simulink model "A3VSM390_2023b"  (R2023b)
settings: Solver=ode14x  StartTime=0  StopTime=Sim.tend  FixedStep=0.000125  RelTol=4e-4
values from neighbouring files (symbols this model uses):
  center_line_status = parameterset.center_line_status    [sim3run_390.m]
  ControlSampleTime = 1/8000    (= 0.000125)    [sim3run_390.m]
  k_ring1 = 1    [sim3run_390.m]
  k_ring2 = 1    [sim3run_390.m]
  load_start_factor = 1    [prm3var_390.m]    (also in simu3_826.m = 0.9; simu3_827.m = 0.9)
  lower_line_status = parameterset.lower_line_status    [sim3run_390.m]
  mZC = 3    [sim3run_390.m]
undefined symbols (not defined in the file or in its folder): Event, General, InfBus, Li, parameterset, prm_vsm, pu_vsm, TrG, VSM
libraries: fl_lib x92, nesl_utility x69, ee_lib x36, spsPower3phInstantaneousLib x5, simulink x2, eeTransforms x1
(part 2 of 3)

== system A3VSM390_2023b/Inverter AverageMdl LC SimScape0/Modul F30 fixed DC voltage Average SimScape ==
  ctrl : Inport
  Phase Splitter : ee_lib/Connectors & References/Phase Splitter
  Rate Transition : RateTransition  Integrity=off  InitialCondition=-1  OutPortSampleTime=ControlSampleTime
  ctrlSelect3 : Subsystem
  measMerge3 : Subsystem
  simscape_bridgefilter_aca : Subsystem  mask{L1=L1, R_L1=R_L1, C1=C1, R_C1=R_C1}
      mask prompts: L1 "Inductance L1 [H]"; R_L1 "Resistance of L1 [Ohm]"; C1 "Capacitance C1 [F]"; R_C1 "Parallel resistance of C1 [Ohm]"
      mask DialogControl LC Prompt: LC(L)(C)
      mask DialogControl GrpLC Prompt: LC(L)(C)-Filter
  simscape_bridgefilter_aca1 : Subsystem  mask{L1=L1, R_L1=R_L1, C1=C1, R_C1=R_C1}
      mask prompts: L1 "Inductance L1 [H]"; R_L1 "Resistance of L1 [Ohm]"; C1 "Capacitance C1 [F]"; R_C1 "Parallel resistance of C1 [Ohm]"
      mask DialogControl LC Prompt: LC(L)(C)
      mask DialogControl GrpLC Prompt: LC(L)(C)-Filter
  simscape_bridgefilter_aca2 : Subsystem  mask{L1=L1, R_L1=R_L1, C1=C1, R_C1=R_C1}
      mask prompts: L1 "Inductance L1 [H]"; R_L1 "Resistance of L1 [Ohm]"; C1 "Capacitance C1 [F]"; R_C1 "Parallel resistance of C1 [Ohm]"
      mask DialogControl LC Prompt: LC(L)(C)
      mask DialogControl GrpLC Prompt: LC(L)(C)-Filter
  N : PMIOPort  Side=Left
  ABC : PMIOPort  Port=2  Side=Right
  meas : Outport  VectorParamsAs1DForOutWhenUnconnected=off
  wires:
  measMerge3/1(meas) -> Rate Transition/1
  ctrlSelect3/1(ctrl1) -> simscape_bridgefilter_aca/1(ctrl)
  [ctrl3] -> simscape_bridgefilter_aca2/1(ctrl)
  [ctrl2] -> simscape_bridgefilter_aca1/1(ctrl)
  ctrlSelect3/2(ctrl2) -> [ctrl2]
  ctrlSelect3/3(ctrl3) -> [ctrl3]
  ctrl/1 -> ctrlSelect3/1(ctrl)
  [meas2] -> measMerge3/2(meas2)
  simscape_bridgefilter_aca2/1(meas) -> [meas3]
  simscape_bridgefilter_aca1/1(meas) -> [meas2]
  [meas3] -> measMerge3/3(meas3)
  simscape_bridgefilter_aca/1(meas) -> measMerge3/1(meas1)
  Rate Transition/1 -> meas/1
  connections:
  simscape_bridgefilter_aca/LConn2 -- simscape_bridgefilter_aca1/LConn2 -- simscape_bridgefilter_aca2/LConn2 -- N/RConn1
  simscape_bridgefilter_aca/RConn1 -- simscape_bridgefilter_aca2/RConn1 -- simscape_bridgefilter_aca1/RConn1
  simscape_bridgefilter_aca2/LConn1 -- Phase Splitter/RConn3
  ABC/RConn1 -- Phase Splitter/LConn1
  Phase Splitter/RConn1 -- simscape_bridgefilter_aca/LConn1
  simscape_bridgefilter_aca1/LConn1 -- Phase Splitter/RConn2

== system A3VSM390_2023b/Inverter AverageMdl LC SimScape1/Modul F30 fixed DC voltage Average SimScape ==
  ctrl : Inport
  Phase Splitter : ee_lib/Connectors & References/Phase Splitter
  Rate Transition : RateTransition  Integrity=off  InitialCondition=-1  OutPortSampleTime=ControlSampleTime
  ctrlSelect3 : Subsystem
  measMerge3 : Subsystem
  simscape_bridgefilter_aca : Subsystem  mask{L1=L1, R_L1=R_L1, C1=C1, R_C1=R_C1}
      mask prompts: L1 "Inductance L1 [H]"; R_L1 "Resistance of L1 [Ohm]"; C1 "Capacitance C1 [F]"; R_C1 "Parallel resistance of C1 [Ohm]"
      mask DialogControl LC Prompt: LC(L)(C)
      mask DialogControl GrpLC Prompt: LC(L)(C)-Filter
  simscape_bridgefilter_aca1 : Subsystem  mask{L1=L1, R_L1=R_L1, C1=C1, R_C1=R_C1}
      mask prompts: L1 "Inductance L1 [H]"; R_L1 "Resistance of L1 [Ohm]"; C1 "Capacitance C1 [F]"; R_C1 "Parallel resistance of C1 [Ohm]"
      mask DialogControl LC Prompt: LC(L)(C)
      mask DialogControl GrpLC Prompt: LC(L)(C)-Filter
  simscape_bridgefilter_aca2 : Subsystem  mask{L1=L1, R_L1=R_L1, C1=C1, R_C1=R_C1}
      mask prompts: L1 "Inductance L1 [H]"; R_L1 "Resistance of L1 [Ohm]"; C1 "Capacitance C1 [F]"; R_C1 "Parallel resistance of C1 [Ohm]"
      mask DialogControl LC Prompt: LC(L)(C)
      mask DialogControl GrpLC Prompt: LC(L)(C)-Filter
  N : PMIOPort  Side=Left
  ABC : PMIOPort  Port=2  Side=Right
  meas : Outport  VectorParamsAs1DForOutWhenUnconnected=off
  wires:
  measMerge3/1(meas) -> Rate Transition/1
  ctrlSelect3/1(ctrl1) -> simscape_bridgefilter_aca/1(ctrl)
  [ctrl3] -> simscape_bridgefilter_aca2/1(ctrl)
  [ctrl2] -> simscape_bridgefilter_aca1/1(ctrl)
  ctrlSelect3/2(ctrl2) -> [ctrl2]
  ctrlSelect3/3(ctrl3) -> [ctrl3]
  ctrl/1 -> ctrlSelect3/1(ctrl)
  [meas2] -> measMerge3/2(meas2)
  simscape_bridgefilter_aca2/1(meas) -> [meas3]
  simscape_bridgefilter_aca1/1(meas) -> [meas2]
  [meas3] -> measMerge3/3(meas3)
  simscape_bridgefilter_aca/1(meas) -> measMerge3/1(meas1)
  Rate Transition/1 -> meas/1
  connections:
  simscape_bridgefilter_aca/LConn2 -- simscape_bridgefilter_aca1/LConn2 -- simscape_bridgefilter_aca2/LConn2 -- N/RConn1
  simscape_bridgefilter_aca/RConn1 -- simscape_bridgefilter_aca2/RConn1 -- simscape_bridgefilter_aca1/RConn1
  simscape_bridgefilter_aca2/LConn1 -- Phase Splitter/RConn3
  ABC/RConn1 -- Phase Splitter/LConn1
  Phase Splitter/RConn1 -- simscape_bridgefilter_aca/LConn1
  simscape_bridgefilter_aca1/LConn1 -- Phase Splitter/RConn2

== system A3VSM390_2023b/Inverter AverageMdl LC SimScape2/Modul F30 fixed DC voltage Average SimScape ==
  ctrl : Inport
  Phase Splitter : ee_lib/Connectors & References/Phase Splitter
  Rate Transition : RateTransition  Integrity=off  InitialCondition=-1  OutPortSampleTime=ControlSampleTime
  ctrlSelect3 : Subsystem
  measMerge3 : Subsystem
  simscape_bridgefilter_aca : Subsystem  mask{L1=L1, R_L1=R_L1, C1=C1, R_C1=R_C1}
      mask prompts: L1 "Inductance L1 [H]"; R_L1 "Resistance of L1 [Ohm]"; C1 "Capacitance C1 [F]"; R_C1 "Parallel resistance of C1 [Ohm]"
      mask DialogControl LC Prompt: LC(L)(C)
      mask DialogControl GrpLC Prompt: LC(L)(C)-Filter
  simscape_bridgefilter_aca1 : Subsystem  mask{L1=L1, R_L1=R_L1, C1=C1, R_C1=R_C1}
      mask prompts: L1 "Inductance L1 [H]"; R_L1 "Resistance of L1 [Ohm]"; C1 "Capacitance C1 [F]"; R_C1 "Parallel resistance of C1 [Ohm]"
      mask DialogControl LC Prompt: LC(L)(C)
      mask DialogControl GrpLC Prompt: LC(L)(C)-Filter
  simscape_bridgefilter_aca2 : Subsystem  mask{L1=L1, R_L1=R_L1, C1=C1, R_C1=R_C1}
      mask prompts: L1 "Inductance L1 [H]"; R_L1 "Resistance of L1 [Ohm]"; C1 "Capacitance C1 [F]"; R_C1 "Parallel resistance of C1 [Ohm]"
      mask DialogControl LC Prompt: LC(L)(C)
      mask DialogControl GrpLC Prompt: LC(L)(C)-Filter
  N : PMIOPort  Side=Left
  ABC : PMIOPort  Port=2  Side=Right
  meas : Outport  VectorParamsAs1DForOutWhenUnconnected=off
  wires:
  measMerge3/1(meas) -> Rate Transition/1
  ctrlSelect3/1(ctrl1) -> simscape_bridgefilter_aca/1(ctrl)
  [ctrl3] -> simscape_bridgefilter_aca2/1(ctrl)
  [ctrl2] -> simscape_bridgefilter_aca1/1(ctrl)
  ctrlSelect3/2(ctrl2) -> [ctrl2]
  ctrlSelect3/3(ctrl3) -> [ctrl3]
  ctrl/1 -> ctrlSelect3/1(ctrl)
  [meas2] -> measMerge3/2(meas2)
  simscape_bridgefilter_aca2/1(meas) -> [meas3]
  simscape_bridgefilter_aca1/1(meas) -> [meas2]
  [meas3] -> measMerge3/3(meas3)
  simscape_bridgefilter_aca/1(meas) -> measMerge3/1(meas1)
  Rate Transition/1 -> meas/1
  connections:
  simscape_bridgefilter_aca/LConn2 -- simscape_bridgefilter_aca1/LConn2 -- simscape_bridgefilter_aca2/LConn2 -- N/RConn1
  simscape_bridgefilter_aca/RConn1 -- simscape_bridgefilter_aca2/RConn1 -- simscape_bridgefilter_aca1/RConn1
  simscape_bridgefilter_aca2/LConn1 -- Phase Splitter/RConn3
  ABC/RConn1 -- Phase Splitter/LConn1
  Phase Splitter/RConn1 -- simscape_bridgefilter_aca/LConn1
  simscape_bridgefilter_aca1/LConn1 -- Phase Splitter/RConn2

== system A3VSM390_2023b/Subsystem2/I_PhN1 ==
  In1 : Inport
  Abs : Abs  SaturateOnIntegerOverflow=off
  Demux : Demux  Outputs=2
  PhN->ab0 : Subsystem
      mask Display:
      | plot([0 1], [0,1])
      | plot([0.1 0.25 0.4 0.25 0.25], [0.5 0.6 0.5 0.6 0.8]) % Stern
      | text(0.05,1,'PhN','VerticalAlignment','Top')
      | text(0.55, 0.3,'\alpha\beta0','texmode','on')
  Real-Imag to Complex : RealImagToComplex
  Selector4 : Selector  InputPortWidth=3  IndexOptions=Index vector (dialog)  Indices=[1 2]  OutputSizes=1
  Out1 : Outport  VectorParamsAs1DForOutWhenUnconnected=off
  wires:
  Demux/1 -> Real-Imag to Complex/1
  PhN->ab0/1(ab0) -> Selector4/1
  Selector4/1 -> Demux/1
  Real-Imag to Complex/1 -> Abs/1
  Demux/2 -> Real-Imag to Complex/2
  Abs/1 -> Out1/1
  In1/1 -> PhN->ab0/1(PhN)

== system A3VSM390_2023b/Subsystem2/I_PhN2 ==
  In1 : Inport
  Abs : Abs  SaturateOnIntegerOverflow=off
  Demux : Demux  Outputs=2
  PhN->ab0 : Subsystem
      mask Display:
      | plot([0 1], [0,1])
      | plot([0.1 0.25 0.4 0.25 0.25], [0.5 0.6 0.5 0.6 0.8]) % Stern
      | text(0.05,1,'PhN','VerticalAlignment','Top')
      | text(0.55, 0.3,'\alpha\beta0','texmode','on')
  Real-Imag to Complex : RealImagToComplex
  Selector4 : Selector  InputPortWidth=3  IndexOptions=Index vector (dialog)  Indices=[1 2]  OutputSizes=1
  Out1 : Outport  VectorParamsAs1DForOutWhenUnconnected=off
  wires:
  Demux/1 -> Real-Imag to Complex/1
  PhN->ab0/1(ab0) -> Selector4/1
  Selector4/1 -> Demux/1
  Real-Imag to Complex/1 -> Abs/1
  Demux/2 -> Real-Imag to Complex/2
  Abs/1 -> Out1/1
  In1/1 -> PhN->ab0/1(PhN)

== system A3VSM390_2023b/Subsystem2/I_PhN3 ==
  In1 : Inport
  Abs : Abs  SaturateOnIntegerOverflow=off
  Demux : Demux  Outputs=2
  PhN->ab0 : Subsystem
      mask Display:
      | plot([0 1], [0,1])
      | plot([0.1 0.25 0.4 0.25 0.25], [0.5 0.6 0.5 0.6 0.8]) % Stern
      | text(0.05,1,'PhN','VerticalAlignment','Top')
      | text(0.55, 0.3,'\alpha\beta0','texmode','on')
  Real-Imag to Complex : RealImagToComplex
  Selector4 : Selector  InputPortWidth=3  IndexOptions=Index vector (dialog)  Indices=[1 2]  OutputSizes=1
  Out1 : Outport  VectorParamsAs1DForOutWhenUnconnected=off
  wires:
  Demux/1 -> Real-Imag to Complex/1
  PhN->ab0/1(ab0) -> Selector4/1
  Selector4/1 -> Demux/1
  Real-Imag to Complex/1 -> Abs/1
  Demux/2 -> Real-Imag to Complex/2
  Abs/1 -> Out1/1
  In1/1 -> PhN->ab0/1(PhN)

== system A3VSM390_2023b/Subsystem2/I_PhN4 ==
  In1 : Inport
  Abs : Abs  SaturateOnIntegerOverflow=off
  Demux : Demux  Outputs=2
  PhN->ab0 : Subsystem
      mask Display:
      | plot([0 1], [0,1])
      | plot([0.1 0.25 0.4 0.25 0.25], [0.5 0.6 0.5 0.6 0.8]) % Stern
      | text(0.05,1,'PhN','VerticalAlignment','Top')
      | text(0.55, 0.3,'\alpha\beta0','texmode','on')
  Real-Imag to Complex : RealImagToComplex
  Selector4 : Selector  InputPortWidth=3  IndexOptions=Index vector (dialog)  Indices=[1 2]  OutputSizes=1
  Out1 : Outport  VectorParamsAs1DForOutWhenUnconnected=off
  wires:
  In1/1 -> PhN->ab0/1(PhN)
  Abs/1 -> Out1/1
  Demux/2 -> Real-Imag to Complex/2
  Real-Imag to Complex/1 -> Abs/1
  Selector4/1 -> Demux/1
  PhN->ab0/1(ab0) -> Selector4/1
  Demux/1 -> Real-Imag to Complex/1

== system A3VSM390_2023b/Subsystem2/I_PhN5 ==
  In1 : Inport
  Abs : Abs  SaturateOnIntegerOverflow=off
  Demux : Demux  Outputs=2
  PhN->ab0 : Subsystem
      mask Display:
      | plot([0 1], [0,1])
      | plot([0.1 0.25 0.4 0.25 0.25], [0.5 0.6 0.5 0.6 0.8]) % Stern
      | text(0.05,1,'PhN','VerticalAlignment','Top')
      | text(0.55, 0.3,'\alpha\beta0','texmode','on')
  Real-Imag to Complex : RealImagToComplex
  Selector4 : Selector  InputPortWidth=3  IndexOptions=Index vector (dialog)  Indices=[1 2]  OutputSizes=1
  Out1 : Outport  VectorParamsAs1DForOutWhenUnconnected=off
  wires:
  Demux/1 -> Real-Imag to Complex/1
  PhN->ab0/1(ab0) -> Selector4/1
  Selector4/1 -> Demux/1
  Real-Imag to Complex/1 -> Abs/1
  Demux/2 -> Real-Imag to Complex/2
  Abs/1 -> Out1/1
  In1/1 -> PhN->ab0/1(PhN)

== system A3VSM390_2023b/Subsystem2/V_PhN ==
  In1 : Inport
  Abs : Abs  SaturateOnIntegerOverflow=off
  Demux : Demux  Outputs=2
  PhN->ab0 : Subsystem
      mask Display:
      | plot([0 1], [0,1])
      | plot([0.1 0.25 0.4 0.25 0.25], [0.5 0.6 0.5 0.6 0.8]) % Stern
      | text(0.05,1,'PhN','VerticalAlignment','Top')
      | text(0.55, 0.3,'\alpha\beta0','texmode','on')
  Real-Imag to Complex : RealImagToComplex
  Selector4 : Selector  InputPortWidth=3  IndexOptions=Index vector (dialog)  Indices=[1 2]  OutputSizes=1
  Out1 : Outport  VectorParamsAs1DForOutWhenUnconnected=off
  wires:
  In1/1 -> PhN->ab0/1(PhN)
  Abs/1 -> Out1/1
  Demux/2 -> Real-Imag to Complex/2
  Real-Imag to Complex/1 -> Abs/1
  Selector4/1 -> Demux/1
  PhN->ab0/1(ab0) -> Selector4/1
  Demux/1 -> Real-Imag to Complex/1

== system A3VSM390_2023b/Subsystem2/V_PhN1 ==
  In1 : Inport
  Abs : Abs  SaturateOnIntegerOverflow=off
  Demux : Demux  Outputs=2
  PhN->ab0 : Subsystem
      mask Display:
      | plot([0 1], [0,1])
      | plot([0.1 0.25 0.4 0.25 0.25], [0.5 0.6 0.5 0.6 0.8]) % Stern
      | text(0.05,1,'PhN','VerticalAlignment','Top')
      | text(0.55, 0.3,'\alpha\beta0','texmode','on')
  Real-Imag to Complex : RealImagToComplex
  Selector4 : Selector  InputPortWidth=3  IndexOptions=Index vector (dialog)  Indices=[1 2]  OutputSizes=1
  Out1 : Outport  VectorParamsAs1DForOutWhenUnconnected=off
  wires:
  Demux/1 -> Real-Imag to Complex/1
  PhN->ab0/1(ab0) -> Selector4/1
  Selector4/1 -> Demux/1
  Real-Imag to Complex/1 -> Abs/1
  Demux/2 -> Real-Imag to Complex/2
  Abs/1 -> Out1/1
  In1/1 -> PhN->ab0/1(PhN)

== system A3VSM390_2023b/Subsystem2/V_PhN2 ==
  In1 : Inport
  Abs : Abs  SaturateOnIntegerOverflow=off
  Demux : Demux  Outputs=2
  PhN->ab0 : Subsystem
      mask Display:
      | plot([0 1], [0,1])
      | plot([0.1 0.25 0.4 0.25 0.25], [0.5 0.6 0.5 0.6 0.8]) % Stern
      | text(0.05,1,'PhN','VerticalAlignment','Top')
      | text(0.55, 0.3,'\alpha\beta0','texmode','on')
  Real-Imag to Complex : RealImagToComplex
  Selector4 : Selector  InputPortWidth=3  IndexOptions=Index vector (dialog)  Indices=[1 2]  OutputSizes=1
  Out1 : Outport  VectorParamsAs1DForOutWhenUnconnected=off
  wires:
  Demux/1 -> Real-Imag to Complex/1
  PhN->ab0/1(ab0) -> Selector4/1
  Selector4/1 -> Demux/1
  Real-Imag to Complex/1 -> Abs/1
  Demux/2 -> Real-Imag to Complex/2
  Abs/1 -> Out1/1
  In1/1 -> PhN->ab0/1(PhN)

== system A3VSM390_2023b/Subsystem2/V_PhN3 ==
  In1 : Inport
  Abs : Abs  SaturateOnIntegerOverflow=off
  Demux : Demux  Outputs=2
  PhN->ab0 : Subsystem
      mask Display:
      | plot([0 1], [0,1])
      | plot([0.1 0.25 0.4 0.25 0.25], [0.5 0.6 0.5 0.6 0.8]) % Stern
      | text(0.05,1,'PhN','VerticalAlignment','Top')
      | text(0.55, 0.3,'\alpha\beta0','texmode','on')
  Real-Imag to Complex : RealImagToComplex
  Selector4 : Selector  InputPortWidth=3  IndexOptions=Index vector (dialog)  Indices=[1 2]  OutputSizes=1
  Out1 : Outport  VectorParamsAs1DForOutWhenUnconnected=off
  wires:
  Demux/1 -> Real-Imag to Complex/1
  PhN->ab0/1(ab0) -> Selector4/1
  Selector4/1 -> Demux/1
  Real-Imag to Complex/1 -> Abs/1
  Demux/2 -> Real-Imag to Complex/2
  Abs/1 -> Out1/1
  In1/1 -> PhN->ab0/1(PhN)

== system A3VSM390_2023b/Subsystem2/V_PhN4 ==
  In1 : Inport
  Abs : Abs  SaturateOnIntegerOverflow=off
  Demux : Demux  Outputs=2
  PhN->ab0 : Subsystem
      mask Display:
      | plot([0 1], [0,1])
      | plot([0.1 0.25 0.4 0.25 0.25], [0.5 0.6 0.5 0.6 0.8]) % Stern
      | text(0.05,1,'PhN','VerticalAlignment','Top')
      | text(0.55, 0.3,'\alpha\beta0','texmode','on')
  Real-Imag to Complex : RealImagToComplex
  Selector4 : Selector  InputPortWidth=3  IndexOptions=Index vector (dialog)  Indices=[1 2]  OutputSizes=1
  Out1 : Outport  VectorParamsAs1DForOutWhenUnconnected=off
  wires:
  Demux/1 -> Real-Imag to Complex/1
  PhN->ab0/1(ab0) -> Selector4/1
  Selector4/1 -> Demux/1
  Real-Imag to Complex/1 -> Abs/1
  Demux/2 -> Real-Imag to Complex/2
  Abs/1 -> Out1/1
  In1/1 -> PhN->ab0/1(PhN)

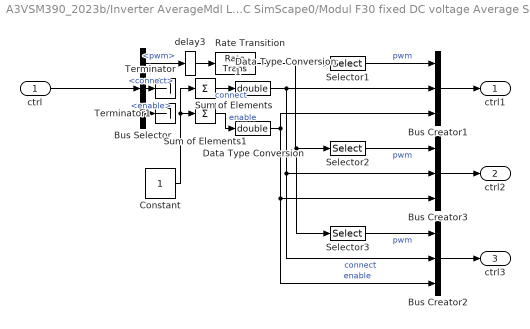
== system A3VSM390_2023b/Inverter AverageMdl LC SimScape0/Modul F30 fixed DC voltage Average SimScape/ctrlSelect3 ==
  ctrl : Inport
  Bus Creator1 : BusCreator  Inputs=3
  Bus Creator2 : BusCreator  Inputs=3
  Bus Creator3 : BusCreator  Inputs=3
  Bus Selector : BusSelector  OutputSignals=pwm,connect,enable
  Constant : Constant
  Data Type Conversion : DataTypeConversion  OutDataTypeStr=double  SaturateOnIntegerOverflow=off  RndMeth=Floor
  Data Type Conversion1 : DataTypeConversion  OutDataTypeStr=double  SaturateOnIntegerOverflow=off  RndMeth=Floor
  Rate Transition : RateTransition  Integrity=off  Deterministic=off  OutPortSampleTime=0
  Selector1 : Selector  InputPortWidth=3  IndexOptions=Index vector (dialog)  Indices=[1]  OutputSizes=1
  Selector2 : Selector  InputPortWidth=3  IndexOptions=Index vector (dialog)  Indices=2  OutputSizes=1
  Selector3 : Selector  InputPortWidth=3  IndexOptions=Index vector (dialog)  Indices=3  OutputSizes=1
  Sum of Elements : Sum  Inputs=+
  Sum of Elements1 : Sum  Inputs=+  SampleTime=ControlSampleTime
  Terminator : Terminator
  Terminator1 : Terminator
  delay3 : UnitDelay  SampleTime=-1  HasFrameUpgradeWarning=on
  ctrl1 : Outport  VectorParamsAs1DForOutWhenUnconnected=off
  ctrl2 : Outport  Port=2  VectorParamsAs1DForOutWhenUnconnected=off
  ctrl3 : Outport  Port=3  VectorParamsAs1DForOutWhenUnconnected=off
  wires:
  Rate Transition/1 -> Selector1/1, Selector3/1, Selector2/1
  Sum of Elements1/1 -> Data Type Conversion/1  "enable"
  Selector1/1 -> Bus Creator1/1  "pwm"
  Bus Creator3/1 -> ctrl2/1
  Selector2/1 -> Bus Creator3/1  "pwm"
  Sum of Elements/1 -> Data Type Conversion1/1  "connect"
  Bus Creator1/1 -> ctrl1/1
  ctrl/1 -> Bus Selector/1
  Bus Creator2/1 -> ctrl3/1
  Selector3/1 -> Bus Creator2/1  "pwm"
  Bus Selector/1 -> delay3/1  "<pwm>"
  Data Type Conversion/1 -> Bus Creator1/3, Bus Creator2/3, Bus Creator3/3  "enable"
  Data Type Conversion1/1 -> Bus Creator2/2, Bus Creator3/2, Bus Creator1/2  "connect"
  Constant/1 -> Sum of Elements1/1, Sum of Elements/1
  Bus Selector/2 -> Terminator/1  "<connect>"
  Bus Selector/3 -> Terminator1/1  "<enable>"
  delay3/1 -> Rate Transition/1

== system A3VSM390_2023b/Inverter AverageMdl LC SimScape0/Modul F30 fixed DC voltage Average SimScape/measMerge3 ==
  meas1 : Inport
  meas2 : Inport  Port=2
  meas3 : Inport  Port=3
  measMerge123 : Subsystem
  meas : Outport  VectorParamsAs1DForOutWhenUnconnected=off
  wires:
  meas3/1 -> measMerge123/3(meas3)
  meas2/1 -> measMerge123/2(meas2)
  measMerge123/1(meas) -> meas/1
  meas1/1 -> measMerge123/1(meas1)

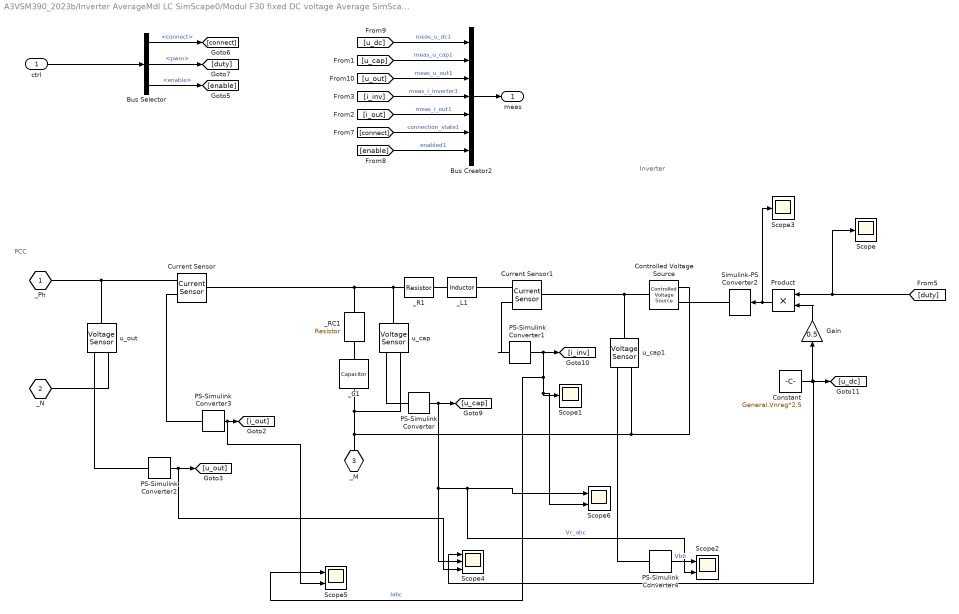
== system A3VSM390_2023b/Inverter AverageMdl LC SimScape0/Modul F30 fixed DC voltage Average SimScape/simscape_bridgefilter_aca ==
  note: Inverter
  note: PCC
  ctrl : Inport
  Bus Creator2 : BusCreator  Inputs=7
  Bus Selector : BusSelector  OutputSignals=connect,pwm,enable
  Constant : Constant  Value=General.Vnreg*2.5
  Controlled Voltage Source : fl_lib/Electrical/Electrical Sources/Controlled Voltage Source
  Current Sensor : fl_lib/Electrical/Electrical Sensors/Current Sensor
  Current Sensor1 : fl_lib/Electrical/Electrical Sensors/Current Sensor
  Gain : Gain  Gain=0.5
  PS-Simulink Converter{,1..4} (5 alike) : nesl_utility/PS-Simulink Converter  PhysicalDomain=network_engine_domain  SubClassName=ps_output  LeftPortType=input  RightPortType=output  PseudoPeriodic=off  Frequencies=[]  VectorFormat=1-D array  Unit=1  AffineConversion=off
  Product : Product
  Scope : Scope
  Scope1 : Scope
  Scope2 : Scope  NumInputPorts=2
  Scope3 : Scope
  Scope4 : Scope  NumInputPorts=3
  Scope5 : Scope  NumInputPorts=2
  Scope6 : Scope  NumInputPorts=2
  Simulink-PS Converter2 : nesl_utility/Simulink-PS Converter  PhysicalDomain=network_engine_domain  SubClassName=ps_input  LeftPortType=input  RightPortType=output  PseudoPeriodic=off  Frequencies=[]  NoiseDistribution=none  NoiseParameters=[]  Unit=1  AffineConversion=off  FilteringAndDerivatives=zero  SimscapeFilterOrder=1  InputFilterTimeConstant=0.001  UdotUserProvided=1
  _C1 : fl_lib/Electrical/Electrical Elements/Capacitor  c=C1 F  r=1e-6 Ohm  g=0 1/Ohm  i_specify=off  i_priority=None  i=0 A  i_nominal_specify=off  i_nominal_unit=A  i_nominal_value=1  v_specify=off  v_priority=None  v=0 V  v_nominal_specify=off  v_nominal_unit=V  v_nominal_value=1  vc_specify=off  vc_priority=None  vc=0 V  vc_nominal_specify=off  vc_nominal_unit=V  vc_nominal_value=1
  _L1 : fl_lib/Electrical/Electrical Elements/Inductor  l=L1 H  r=0 Ohm  g=1e-9 1/Ohm  i_specify=off  i_priority=None  i=0 A  i_nominal_specify=off  i_nominal_unit=A  i_nominal_value=1  v_specify=off  v_priority=None  v=0 V  v_nominal_specify=off  v_nominal_unit=V  v_nominal_value=1  i_L_specify=off  i_L_priority=None  i_L=0 A  i_L_nominal_specify=off  i_L_nominal_unit=A  i_L_nominal_value=1
  _R1 : fl_lib/Electrical/Electrical Elements/Resistor  R=R_L1 Ohm  i_specify=off  i_priority=None  i=0 A  i_nominal_specify=off  i_nominal_unit=A  i_nominal_value=1  v_specify=off  v_priority=None  v=0 V  v_nominal_specify=off  v_nominal_unit=V  v_nominal_value=1
  _RC1 : fl_lib/Electrical/Electrical Elements/Resistor  R=R_C1 Ohm  i_specify=off  i_priority=None  i=0 A  i_nominal_specify=off  i_nominal_unit=A  i_nominal_value=1  v_specify=off  v_priority=None  v=0 V  v_nominal_specify=off  v_nominal_unit=V  v_nominal_value=1
  u_cap : fl_lib/Electrical/Electrical Sensors/Voltage Sensor
  u_cap1 : fl_lib/Electrical/Electrical Sensors/Voltage Sensor
  u_out : fl_lib/Electrical/Electrical Sensors/Voltage Sensor
  _Ph : PMIOPort  Side=Left
  _N : PMIOPort  Port=2  Side=Left
  _M : PMIOPort  Port=3  Side=Right
  meas : Outport  VectorParamsAs1DForOutWhenUnconnected=off
  wires:
  Bus Selector/2 -> [duty]  "<pwm>"
  Bus Selector/1 -> [connect]  "<connect>"
  [connect] -> Bus Creator2/6  "connection_state1"
  ctrl/1 -> Bus Selector/1
  [i_out] -> Bus Creator2/5  "meas_i_out1"
  [i_inv] -> Bus Creator2/4  "meas_i_inverter1"
  [u_out] -> Bus Creator2/3  "meas_u_out1"
  [u_cap] -> Bus Creator2/2  "meas_u_cap1"
  Bus Selector/3 -> [enable]  "<enable>"
  [enable] -> Bus Creator2/7  "enabled1"
  Bus Creator2/1 -> meas/1
  [u_dc] -> Bus Creator2/1  "meas_u_dc1"
  PS-Simulink Converter/1 -> Scope2/2, Scope6/1, Scope4/2, [u_cap]  "Vc_abc"
  PS-Simulink Converter1/1 -> Scope5/1, Scope6/2, Scope1/1, [i_inv]  "Iabc"
  PS-Simulink Converter2/1 -> Scope4/3, [u_out]
  PS-Simulink Converter3/1 -> Scope5/2, [i_out]
  Product/1 -> Scope3/1, Simulink-PS Converter2/1
  Constant/1 -> Scope4/1, [u_dc], Gain/1
  [duty] -> Scope/1, Product/1
  Gain/1 -> Product/2
  PS-Simulink Converter4/1 -> Scope2/1  "Vb6"
  connections:
  _R1/RConn1 -- _L1/LConn1
  Current Sensor1/RConn2 -- _L1/RConn1
  Current Sensor/LConn1 -- _RC1/LConn1 -- u_cap/LConn1 -- _R1/LConn1
  Controlled Voltage Source/RConn2 -- u_cap1/RConn2 -- _M/RConn1 -- u_cap/RConn2 -- _C1/RConn1
  u_out/LConn1 -- _Ph/RConn1 -- Current Sensor/RConn2
  u_out/RConn2 -- _N/RConn1
  Current Sensor1/LConn1 -- u_cap1/LConn1 -- Controlled Voltage Source/LConn1
  Simulink-PS Converter2/RConn1 -- Controlled Voltage Source/RConn1
  PS-Simulink Converter/LConn1 -- u_cap/RConn1
  PS-Simulink Converter1/LConn1 -- Current Sensor1/RConn1
  PS-Simulink Converter2/LConn1 -- u_out/RConn1
  PS-Simulink Converter3/LConn1 -- Current Sensor/RConn1
  _RC1/RConn1 -- _C1/LConn1
  PS-Simulink Converter4/LConn1 -- u_cap1/RConn1

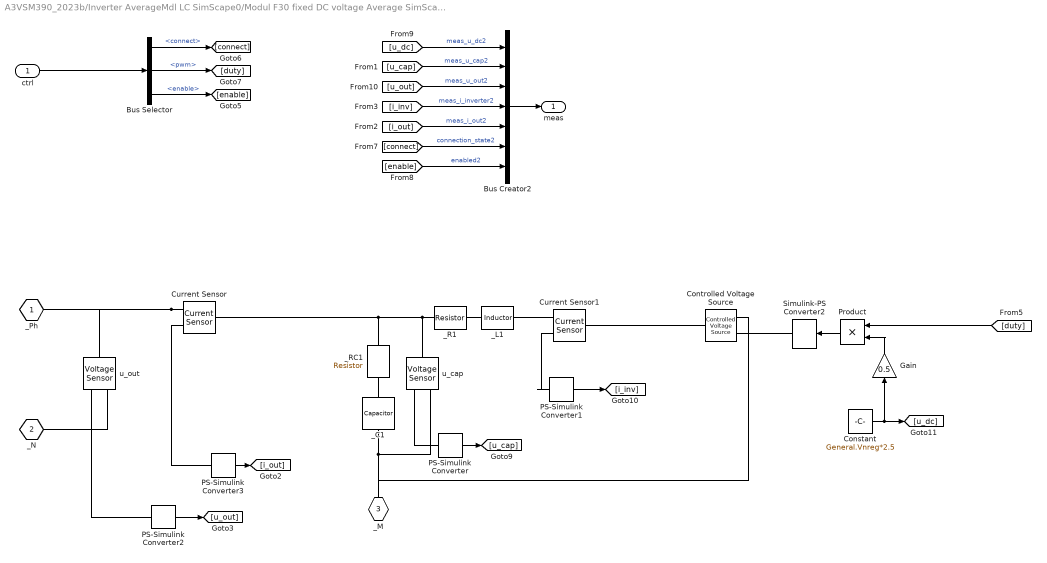
== system A3VSM390_2023b/Inverter AverageMdl LC SimScape0/Modul F30 fixed DC voltage Average SimScape/simscape_bridgefilter_aca1 ==
  ctrl : Inport
  Bus Creator2 : BusCreator  Inputs=7
  Bus Selector : BusSelector  OutputSignals=connect,pwm,enable
  Constant : Constant  Value=General.Vnreg*2.5
  Controlled Voltage Source : fl_lib/Electrical/Electrical Sources/Controlled Voltage Source
  Current Sensor : fl_lib/Electrical/Electrical Sensors/Current Sensor
  Current Sensor1 : fl_lib/Electrical/Electrical Sensors/Current Sensor
  Gain : Gain  Gain=0.5
  PS-Simulink Converter{,1..3} (4 alike) : nesl_utility/PS-Simulink Converter  PhysicalDomain=network_engine_domain  SubClassName=ps_output  LeftPortType=input  RightPortType=output  PseudoPeriodic=off  Frequencies=[]  VectorFormat=1-D array  Unit=1  AffineConversion=off
  Product : Product
  Simulink-PS Converter2 : nesl_utility/Simulink-PS Converter  PhysicalDomain=network_engine_domain  SubClassName=ps_input  LeftPortType=input  RightPortType=output  PseudoPeriodic=off  Frequencies=[]  NoiseDistribution=none  NoiseParameters=[]  Unit=1  AffineConversion=off  FilteringAndDerivatives=zero  SimscapeFilterOrder=1  InputFilterTimeConstant=0.001  UdotUserProvided=1
  _C1 : fl_lib/Electrical/Electrical Elements/Capacitor  c=C1 F  r=1e-6 Ohm  g=0 1/Ohm  i_specify=off  i_priority=None  i=0 A  i_nominal_specify=off  i_nominal_unit=A  i_nominal_value=1  v_specify=off  v_priority=None  v=0 V  v_nominal_specify=off  v_nominal_unit=V  v_nominal_value=1  vc_specify=off  vc_priority=None  vc=0 V  vc_nominal_specify=off  vc_nominal_unit=V  vc_nominal_value=1
  _L1 : fl_lib/Electrical/Electrical Elements/Inductor  l=L1 H  r=0 Ohm  g=1e-9 1/Ohm  i_specify=off  i_priority=None  i=0 A  i_nominal_specify=off  i_nominal_unit=A  i_nominal_value=1  v_specify=off  v_priority=None  v=0 V  v_nominal_specify=off  v_nominal_unit=V  v_nominal_value=1  i_L_specify=off  i_L_priority=None  i_L=0 A  i_L_nominal_specify=off  i_L_nominal_unit=A  i_L_nominal_value=1
  _R1 : fl_lib/Electrical/Electrical Elements/Resistor  R=R_L1 Ohm  i_specify=off  i_priority=None  i=0 A  i_nominal_specify=off  i_nominal_unit=A  i_nominal_value=1  v_specify=off  v_priority=None  v=0 V  v_nominal_specify=off  v_nominal_unit=V  v_nominal_value=1
  _RC1 : fl_lib/Electrical/Electrical Elements/Resistor  R=R_C1 Ohm  i_specify=off  i_priority=None  i=0 A  i_nominal_specify=off  i_nominal_unit=A  i_nominal_value=1  v_specify=off  v_priority=None  v=0 V  v_nominal_specify=off  v_nominal_unit=V  v_nominal_value=1
  u_cap : fl_lib/Electrical/Electrical Sensors/Voltage Sensor
  u_out : fl_lib/Electrical/Electrical Sensors/Voltage Sensor
  _Ph : PMIOPort  Side=Left
  _N : PMIOPort  Port=2  Side=Left
  _M : PMIOPort  Port=3  Side=Right
  meas : Outport  VectorParamsAs1DForOutWhenUnconnected=off
  wires:
  Gain/1 -> Product/2
  [duty] -> Product/1
  Constant/1 -> Gain/1, [u_dc]
  Product/1 -> Simulink-PS Converter2/1
  PS-Simulink Converter3/1 -> [i_out]
  PS-Simulink Converter2/1 -> [u_out]
  PS-Simulink Converter1/1 -> [i_inv]
  PS-Simulink Converter/1 -> [u_cap]
  [u_dc] -> Bus Creator2/1  "meas_u_dc2"
  Bus Creator2/1 -> meas/1
  [enable] -> Bus Creator2/7  "enabled2"
  Bus Selector/3 -> [enable]  "<enable>"
  [u_cap] -> Bus Creator2/2  "meas_u_cap2"
  [u_out] -> Bus Creator2/3  "meas_u_out2"
  [i_inv] -> Bus Creator2/4  "meas_i_inverter2"
  [i_out] -> Bus Creator2/5  "meas_i_out2"
  ctrl/1 -> Bus Selector/1
  [connect] -> Bus Creator2/6  "connection_state2"
  Bus Selector/1 -> [connect]  "<connect>"
  Bus Selector/2 -> [duty]  "<pwm>"
  connections:
  _RC1/RConn1 -- _C1/LConn1
  PS-Simulink Converter3/LConn1 -- Current Sensor/RConn1
  PS-Simulink Converter2/LConn1 -- u_out/RConn1
  PS-Simulink Converter1/LConn1 -- Current Sensor1/RConn1
  PS-Simulink Converter/LConn1 -- u_cap/RConn1
  Simulink-PS Converter2/RConn1 -- Controlled Voltage Source/RConn1
  Current Sensor1/LConn1 -- Controlled Voltage Source/LConn1
  u_out/RConn2 -- _N/RConn1
  Current Sensor/RConn2 -- _Ph/RConn1 -- u_out/LConn1
  _C1/RConn1 -- u_cap/RConn2 -- _M/RConn1 -- Controlled Voltage Source/RConn2
  Current Sensor/LConn1 -- _RC1/LConn1 -- _R1/LConn1 -- u_cap/LConn1
  Current Sensor1/RConn2 -- _L1/RConn1
  _R1/RConn1 -- _L1/LConn1

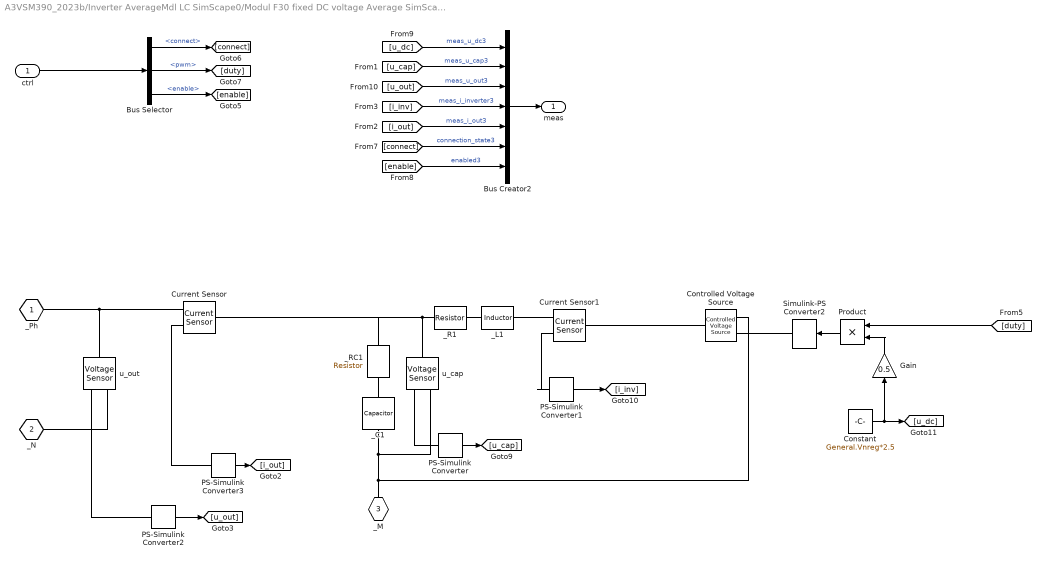
== system A3VSM390_2023b/Inverter AverageMdl LC SimScape0/Modul F30 fixed DC voltage Average SimScape/simscape_bridgefilter_aca2 ==
  ctrl : Inport
  Bus Creator2 : BusCreator  Inputs=7
  Bus Selector : BusSelector  OutputSignals=connect,pwm,enable
  Constant : Constant  Value=General.Vnreg*2.5
  Controlled Voltage Source : fl_lib/Electrical/Electrical Sources/Controlled Voltage Source
  Current Sensor : fl_lib/Electrical/Electrical Sensors/Current Sensor
  Current Sensor1 : fl_lib/Electrical/Electrical Sensors/Current Sensor
  Gain : Gain  Gain=0.5
  PS-Simulink Converter{,1..3} (4 alike) : nesl_utility/PS-Simulink Converter  PhysicalDomain=network_engine_domain  SubClassName=ps_output  LeftPortType=input  RightPortType=output  PseudoPeriodic=off  Frequencies=[]  VectorFormat=1-D array  Unit=1  AffineConversion=off
  Product : Product
  Simulink-PS Converter2 : nesl_utility/Simulink-PS Converter  PhysicalDomain=network_engine_domain  SubClassName=ps_input  LeftPortType=input  RightPortType=output  PseudoPeriodic=off  Frequencies=[]  NoiseDistribution=none  NoiseParameters=[]  Unit=1  AffineConversion=off  FilteringAndDerivatives=zero  SimscapeFilterOrder=1  InputFilterTimeConstant=0.001  UdotUserProvided=1
  _C1 : fl_lib/Electrical/Electrical Elements/Capacitor  c=C1 F  r=1e-6 Ohm  g=0 1/Ohm  i_specify=off  i_priority=None  i=0 A  i_nominal_specify=off  i_nominal_unit=A  i_nominal_value=1  v_specify=off  v_priority=None  v=0 V  v_nominal_specify=off  v_nominal_unit=V  v_nominal_value=1  vc_specify=off  vc_priority=None  vc=0 V  vc_nominal_specify=off  vc_nominal_unit=V  vc_nominal_value=1
  _L1 : fl_lib/Electrical/Electrical Elements/Inductor  l=L1 H  r=0 Ohm  g=1e-9 1/Ohm  i_specify=off  i_priority=None  i=0 A  i_nominal_specify=off  i_nominal_unit=A  i_nominal_value=1  v_specify=off  v_priority=None  v=0 V  v_nominal_specify=off  v_nominal_unit=V  v_nominal_value=1  i_L_specify=off  i_L_priority=None  i_L=0 A  i_L_nominal_specify=off  i_L_nominal_unit=A  i_L_nominal_value=1
  _R1 : fl_lib/Electrical/Electrical Elements/Resistor  R=R_L1 Ohm  i_specify=off  i_priority=None  i=0 A  i_nominal_specify=off  i_nominal_unit=A  i_nominal_value=1  v_specify=off  v_priority=None  v=0 V  v_nominal_specify=off  v_nominal_unit=V  v_nominal_value=1
  _RC1 : fl_lib/Electrical/Electrical Elements/Resistor  R=R_C1 Ohm  i_specify=off  i_priority=None  i=0 A  i_nominal_specify=off  i_nominal_unit=A  i_nominal_value=1  v_specify=off  v_priority=None  v=0 V  v_nominal_specify=off  v_nominal_unit=V  v_nominal_value=1
  u_cap : fl_lib/Electrical/Electrical Sensors/Voltage Sensor
  u_out : fl_lib/Electrical/Electrical Sensors/Voltage Sensor
  _Ph : PMIOPort  Side=Left
  _N : PMIOPort  Port=2  Side=Left
  _M : PMIOPort  Port=3  Side=Right
  meas : Outport  VectorParamsAs1DForOutWhenUnconnected=off
  wires:
  Bus Selector/2 -> [duty]  "<pwm>"
  Bus Selector/1 -> [connect]  "<connect>"
  [connect] -> Bus Creator2/6  "connection_state3"
  ctrl/1 -> Bus Selector/1
  [i_out] -> Bus Creator2/5  "meas_i_out3"
  [i_inv] -> Bus Creator2/4  "meas_i_inverter3"
  [u_out] -> Bus Creator2/3  "meas_u_out3"
  [u_cap] -> Bus Creator2/2  "meas_u_cap3"
  Bus Selector/3 -> [enable]  "<enable>"
  [enable] -> Bus Creator2/7  "enabled3"
  Bus Creator2/1 -> meas/1
  [u_dc] -> Bus Creator2/1  "meas_u_dc3"
  PS-Simulink Converter/1 -> [u_cap]
  PS-Simulink Converter1/1 -> [i_inv]
  PS-Simulink Converter2/1 -> [u_out]
  PS-Simulink Converter3/1 -> [i_out]
  Product/1 -> Simulink-PS Converter2/1
  Constant/1 -> [u_dc], Gain/1
  [duty] -> Product/1
  Gain/1 -> Product/2
  connections:
  _R1/RConn1 -- _L1/LConn1
  Current Sensor1/RConn2 -- _L1/RConn1
  u_cap/LConn1 -- _R1/LConn1 -- _RC1/LConn1 -- Current Sensor/LConn1
  Controlled Voltage Source/RConn2 -- _M/RConn1 -- u_cap/RConn2 -- _C1/RConn1
  u_out/LConn1 -- _Ph/RConn1 -- Current Sensor/RConn2
  u_out/RConn2 -- _N/RConn1
  Current Sensor1/LConn1 -- Controlled Voltage Source/LConn1
  Simulink-PS Converter2/RConn1 -- Controlled Voltage Source/RConn1
  PS-Simulink Converter/LConn1 -- u_cap/RConn1
  PS-Simulink Converter1/LConn1 -- Current Sensor1/RConn1
  PS-Simulink Converter2/LConn1 -- u_out/RConn1
  PS-Simulink Converter3/LConn1 -- Current Sensor/RConn1
  _RC1/RConn1 -- _C1/LConn1

== system A3VSM390_2023b/Inverter AverageMdl LC SimScape1/Modul F30 fixed DC voltage Average SimScape/ctrlSelect3 ==
  ctrl : Inport
  Bus Creator1 : BusCreator  Inputs=3
  Bus Creator2 : BusCreator  Inputs=3
  Bus Creator3 : BusCreator  Inputs=3
  Bus Selector : BusSelector  OutputSignals=pwm,connect,enable
  Constant : Constant
  Data Type Conversion : DataTypeConversion  OutDataTypeStr=double  SaturateOnIntegerOverflow=off  RndMeth=Floor
  Data Type Conversion1 : DataTypeConversion  OutDataTypeStr=double  SaturateOnIntegerOverflow=off  RndMeth=Floor
  Rate Transition : RateTransition  Integrity=off  Deterministic=off  OutPortSampleTime=0
  Selector1 : Selector  InputPortWidth=3  IndexOptions=Index vector (dialog)  Indices=[1]  OutputSizes=1
  Selector2 : Selector  InputPortWidth=3  IndexOptions=Index vector (dialog)  Indices=2  OutputSizes=1
  Selector3 : Selector  InputPortWidth=3  IndexOptions=Index vector (dialog)  Indices=3  OutputSizes=1
  Sum of Elements : Sum  Inputs=+
  Sum of Elements1 : Sum  Inputs=+  SampleTime=ControlSampleTime
  Terminator : Terminator
  Terminator1 : Terminator
  delay3 : UnitDelay  SampleTime=-1  HasFrameUpgradeWarning=on
  ctrl1 : Outport  VectorParamsAs1DForOutWhenUnconnected=off
  ctrl2 : Outport  Port=2  VectorParamsAs1DForOutWhenUnconnected=off
  ctrl3 : Outport  Port=3  VectorParamsAs1DForOutWhenUnconnected=off
  wires:
  Rate Transition/1 -> Selector1/1, Selector3/1, Selector2/1
  Sum of Elements1/1 -> Data Type Conversion/1  "enable"
  Selector1/1 -> Bus Creator1/1  "pwm"
  Bus Creator3/1 -> ctrl2/1
  Selector2/1 -> Bus Creator3/1  "pwm"
  Sum of Elements/1 -> Data Type Conversion1/1  "connect"
  Bus Creator1/1 -> ctrl1/1
  ctrl/1 -> Bus Selector/1
  Bus Creator2/1 -> ctrl3/1
  Selector3/1 -> Bus Creator2/1  "pwm"
  Bus Selector/1 -> delay3/1  "<pwm>"
  Data Type Conversion/1 -> Bus Creator1/3, Bus Creator2/3, Bus Creator3/3  "enable"
  Data Type Conversion1/1 -> Bus Creator2/2, Bus Creator3/2, Bus Creator1/2  "connect"
  Constant/1 -> Sum of Elements1/1, Sum of Elements/1
  Bus Selector/2 -> Terminator/1  "<connect>"
  Bus Selector/3 -> Terminator1/1  "<enable>"
  delay3/1 -> Rate Transition/1

== system A3VSM390_2023b/Inverter AverageMdl LC SimScape1/Modul F30 fixed DC voltage Average SimScape/measMerge3 ==
  meas1 : Inport
  meas2 : Inport  Port=2
  meas3 : Inport  Port=3
  measMerge123 : Subsystem
  meas : Outport  VectorParamsAs1DForOutWhenUnconnected=off
  wires:
  meas3/1 -> measMerge123/3(meas3)
  meas2/1 -> measMerge123/2(meas2)
  measMerge123/1(meas) -> meas/1
  meas1/1 -> measMerge123/1(meas1)

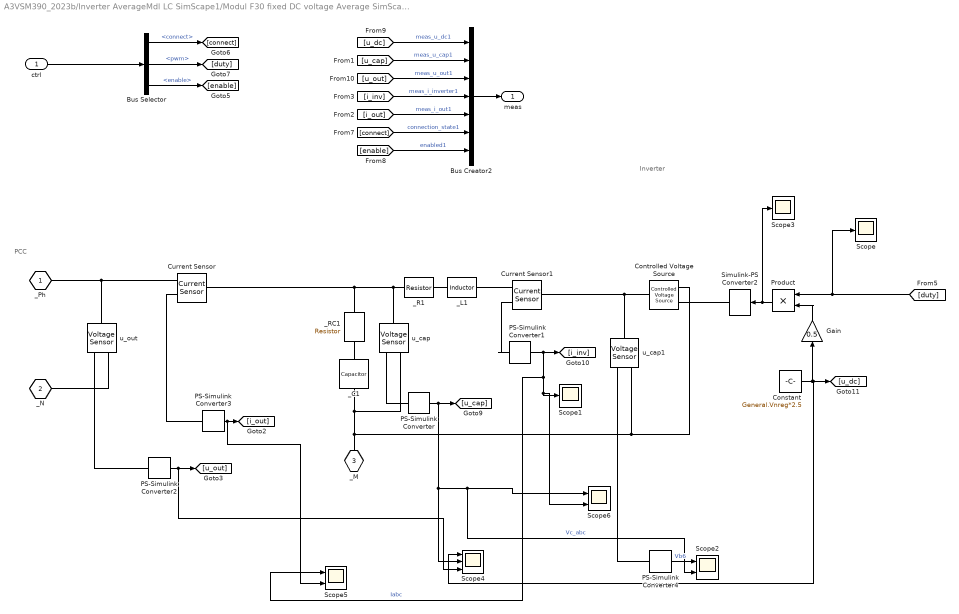
== system A3VSM390_2023b/Inverter AverageMdl LC SimScape1/Modul F30 fixed DC voltage Average SimScape/simscape_bridgefilter_aca ==
  note: Inverter
  note: PCC
  ctrl : Inport
  Bus Creator2 : BusCreator  Inputs=7
  Bus Selector : BusSelector  OutputSignals=connect,pwm,enable
  Constant : Constant  Value=General.Vnreg*2.5
  Controlled Voltage Source : fl_lib/Electrical/Electrical Sources/Controlled Voltage Source
  Current Sensor : fl_lib/Electrical/Electrical Sensors/Current Sensor
  Current Sensor1 : fl_lib/Electrical/Electrical Sensors/Current Sensor
  Gain : Gain  Gain=0.5
  PS-Simulink Converter{,1..4} (5 alike) : nesl_utility/PS-Simulink Converter  PhysicalDomain=network_engine_domain  SubClassName=ps_output  LeftPortType=input  RightPortType=output  PseudoPeriodic=off  Frequencies=[]  VectorFormat=1-D array  Unit=1  AffineConversion=off
  Product : Product
  Scope : Scope
  Scope1 : Scope
  Scope2 : Scope  NumInputPorts=2
  Scope3 : Scope
  Scope4 : Scope  NumInputPorts=3
  Scope5 : Scope  NumInputPorts=2
  Scope6 : Scope  NumInputPorts=2
  Simulink-PS Converter2 : nesl_utility/Simulink-PS Converter  PhysicalDomain=network_engine_domain  SubClassName=ps_input  LeftPortType=input  RightPortType=output  PseudoPeriodic=off  Frequencies=[]  NoiseDistribution=none  NoiseParameters=[]  Unit=1  AffineConversion=off  FilteringAndDerivatives=zero  SimscapeFilterOrder=1  InputFilterTimeConstant=0.001  UdotUserProvided=1
  _C1 : fl_lib/Electrical/Electrical Elements/Capacitor  c=C1 F  r=1e-6 Ohm  g=0 1/Ohm  i_specify=off  i_priority=None  i=0 A  i_nominal_specify=off  i_nominal_unit=A  i_nominal_value=1  v_specify=off  v_priority=None  v=0 V  v_nominal_specify=off  v_nominal_unit=V  v_nominal_value=1  vc_specify=off  vc_priority=None  vc=0 V  vc_nominal_specify=off  vc_nominal_unit=V  vc_nominal_value=1
  _L1 : fl_lib/Electrical/Electrical Elements/Inductor  l=L1 H  r=0 Ohm  g=1e-9 1/Ohm  i_specify=off  i_priority=None  i=0 A  i_nominal_specify=off  i_nominal_unit=A  i_nominal_value=1  v_specify=off  v_priority=None  v=0 V  v_nominal_specify=off  v_nominal_unit=V  v_nominal_value=1  i_L_specify=off  i_L_priority=None  i_L=0 A  i_L_nominal_specify=off  i_L_nominal_unit=A  i_L_nominal_value=1
  _R1 : fl_lib/Electrical/Electrical Elements/Resistor  R=R_L1 Ohm  i_specify=off  i_priority=None  i=0 A  i_nominal_specify=off  i_nominal_unit=A  i_nominal_value=1  v_specify=off  v_priority=None  v=0 V  v_nominal_specify=off  v_nominal_unit=V  v_nominal_value=1
  _RC1 : fl_lib/Electrical/Electrical Elements/Resistor  R=R_C1 Ohm  i_specify=off  i_priority=None  i=0 A  i_nominal_specify=off  i_nominal_unit=A  i_nominal_value=1  v_specify=off  v_priority=None  v=0 V  v_nominal_specify=off  v_nominal_unit=V  v_nominal_value=1
  u_cap : fl_lib/Electrical/Electrical Sensors/Voltage Sensor
  u_cap1 : fl_lib/Electrical/Electrical Sensors/Voltage Sensor
  u_out : fl_lib/Electrical/Electrical Sensors/Voltage Sensor
  _Ph : PMIOPort  Side=Left
  _N : PMIOPort  Port=2  Side=Left
  _M : PMIOPort  Port=3  Side=Right
  meas : Outport  VectorParamsAs1DForOutWhenUnconnected=off
  wires:
  Bus Selector/2 -> [duty]  "<pwm>"
  Bus Selector/1 -> [connect]  "<connect>"
  [connect] -> Bus Creator2/6  "connection_state1"
  ctrl/1 -> Bus Selector/1
  [i_out] -> Bus Creator2/5  "meas_i_out1"
  [i_inv] -> Bus Creator2/4  "meas_i_inverter1"
  [u_out] -> Bus Creator2/3  "meas_u_out1"
  [u_cap] -> Bus Creator2/2  "meas_u_cap1"
  Bus Selector/3 -> [enable]  "<enable>"
  [enable] -> Bus Creator2/7  "enabled1"
  Bus Creator2/1 -> meas/1
  [u_dc] -> Bus Creator2/1  "meas_u_dc1"
  PS-Simulink Converter/1 -> Scope2/2, Scope6/1, Scope4/2, [u_cap]  "Vc_abc"
  PS-Simulink Converter1/1 -> Scope5/1, Scope6/2, Scope1/1, [i_inv]  "Iabc"
  PS-Simulink Converter2/1 -> Scope4/3, [u_out]
  PS-Simulink Converter3/1 -> Scope5/2, [i_out]
  Product/1 -> Scope3/1, Simulink-PS Converter2/1
  Constant/1 -> Scope4/1, [u_dc], Gain/1
  [duty] -> Scope/1, Product/1
  Gain/1 -> Product/2
  PS-Simulink Converter4/1 -> Scope2/1  "Vb6"
  connections:
  _R1/RConn1 -- _L1/LConn1
  Current Sensor1/RConn2 -- _L1/RConn1
  Current Sensor/LConn1 -- _RC1/LConn1 -- u_cap/LConn1 -- _R1/LConn1
  Controlled Voltage Source/RConn2 -- u_cap1/RConn2 -- _M/RConn1 -- u_cap/RConn2 -- _C1/RConn1
  u_out/LConn1 -- _Ph/RConn1 -- Current Sensor/RConn2
  u_out/RConn2 -- _N/RConn1
  Current Sensor1/LConn1 -- u_cap1/LConn1 -- Controlled Voltage Source/LConn1
  Simulink-PS Converter2/RConn1 -- Controlled Voltage Source/RConn1
  PS-Simulink Converter/LConn1 -- u_cap/RConn1
  PS-Simulink Converter1/LConn1 -- Current Sensor1/RConn1
  PS-Simulink Converter2/LConn1 -- u_out/RConn1
  PS-Simulink Converter3/LConn1 -- Current Sensor/RConn1
  _RC1/RConn1 -- _C1/LConn1
  PS-Simulink Converter4/LConn1 -- u_cap1/RConn1

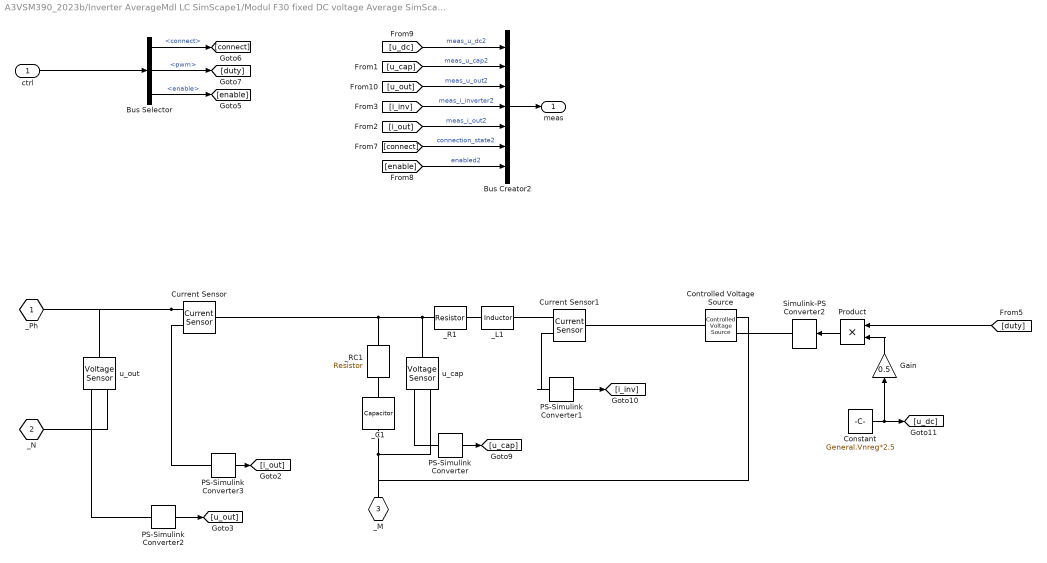
== system A3VSM390_2023b/Inverter AverageMdl LC SimScape1/Modul F30 fixed DC voltage Average SimScape/simscape_bridgefilter_aca1 ==
  ctrl : Inport
  Bus Creator2 : BusCreator  Inputs=7
  Bus Selector : BusSelector  OutputSignals=connect,pwm,enable
  Constant : Constant  Value=General.Vnreg*2.5
  Controlled Voltage Source : fl_lib/Electrical/Electrical Sources/Controlled Voltage Source
  Current Sensor : fl_lib/Electrical/Electrical Sensors/Current Sensor
  Current Sensor1 : fl_lib/Electrical/Electrical Sensors/Current Sensor
  Gain : Gain  Gain=0.5
  PS-Simulink Converter{,1..3} (4 alike) : nesl_utility/PS-Simulink Converter  PhysicalDomain=network_engine_domain  SubClassName=ps_output  LeftPortType=input  RightPortType=output  PseudoPeriodic=off  Frequencies=[]  VectorFormat=1-D array  Unit=1  AffineConversion=off
  Product : Product
  Simulink-PS Converter2 : nesl_utility/Simulink-PS Converter  PhysicalDomain=network_engine_domain  SubClassName=ps_input  LeftPortType=input  RightPortType=output  PseudoPeriodic=off  Frequencies=[]  NoiseDistribution=none  NoiseParameters=[]  Unit=1  AffineConversion=off  FilteringAndDerivatives=zero  SimscapeFilterOrder=1  InputFilterTimeConstant=0.001  UdotUserProvided=1
  _C1 : fl_lib/Electrical/Electrical Elements/Capacitor  c=C1 F  r=1e-6 Ohm  g=0 1/Ohm  i_specify=off  i_priority=None  i=0 A  i_nominal_specify=off  i_nominal_unit=A  i_nominal_value=1  v_specify=off  v_priority=None  v=0 V  v_nominal_specify=off  v_nominal_unit=V  v_nominal_value=1  vc_specify=off  vc_priority=None  vc=0 V  vc_nominal_specify=off  vc_nominal_unit=V  vc_nominal_value=1
  _L1 : fl_lib/Electrical/Electrical Elements/Inductor  l=L1 H  r=0 Ohm  g=1e-9 1/Ohm  i_specify=off  i_priority=None  i=0 A  i_nominal_specify=off  i_nominal_unit=A  i_nominal_value=1  v_specify=off  v_priority=None  v=0 V  v_nominal_specify=off  v_nominal_unit=V  v_nominal_value=1  i_L_specify=off  i_L_priority=None  i_L=0 A  i_L_nominal_specify=off  i_L_nominal_unit=A  i_L_nominal_value=1
  _R1 : fl_lib/Electrical/Electrical Elements/Resistor  R=R_L1 Ohm  i_specify=off  i_priority=None  i=0 A  i_nominal_specify=off  i_nominal_unit=A  i_nominal_value=1  v_specify=off  v_priority=None  v=0 V  v_nominal_specify=off  v_nominal_unit=V  v_nominal_value=1
  _RC1 : fl_lib/Electrical/Electrical Elements/Resistor  R=R_C1 Ohm  i_specify=off  i_priority=None  i=0 A  i_nominal_specify=off  i_nominal_unit=A  i_nominal_value=1  v_specify=off  v_priority=None  v=0 V  v_nominal_specify=off  v_nominal_unit=V  v_nominal_value=1
  u_cap : fl_lib/Electrical/Electrical Sensors/Voltage Sensor
  u_out : fl_lib/Electrical/Electrical Sensors/Voltage Sensor
  _Ph : PMIOPort  Side=Left
  _N : PMIOPort  Port=2  Side=Left
  _M : PMIOPort  Port=3  Side=Right
  meas : Outport  VectorParamsAs1DForOutWhenUnconnected=off
  wires:
  Gain/1 -> Product/2
  [duty] -> Product/1
  Constant/1 -> Gain/1, [u_dc]
  Product/1 -> Simulink-PS Converter2/1
  PS-Simulink Converter3/1 -> [i_out]
  PS-Simulink Converter2/1 -> [u_out]
  PS-Simulink Converter1/1 -> [i_inv]
  PS-Simulink Converter/1 -> [u_cap]
  [u_dc] -> Bus Creator2/1  "meas_u_dc2"
  Bus Creator2/1 -> meas/1
  [enable] -> Bus Creator2/7  "enabled2"
  Bus Selector/3 -> [enable]  "<enable>"
  [u_cap] -> Bus Creator2/2  "meas_u_cap2"
  [u_out] -> Bus Creator2/3  "meas_u_out2"
  [i_inv] -> Bus Creator2/4  "meas_i_inverter2"
  [i_out] -> Bus Creator2/5  "meas_i_out2"
  ctrl/1 -> Bus Selector/1
  [connect] -> Bus Creator2/6  "connection_state2"
  Bus Selector/1 -> [connect]  "<connect>"
  Bus Selector/2 -> [duty]  "<pwm>"
  connections:
  _RC1/RConn1 -- _C1/LConn1
  PS-Simulink Converter3/LConn1 -- Current Sensor/RConn1
  PS-Simulink Converter2/LConn1 -- u_out/RConn1
  PS-Simulink Converter1/LConn1 -- Current Sensor1/RConn1
  PS-Simulink Converter/LConn1 -- u_cap/RConn1
  Simulink-PS Converter2/RConn1 -- Controlled Voltage Source/RConn1
  Current Sensor1/LConn1 -- Controlled Voltage Source/LConn1
  u_out/RConn2 -- _N/RConn1
  Current Sensor/RConn2 -- _Ph/RConn1 -- u_out/LConn1
  _C1/RConn1 -- u_cap/RConn2 -- _M/RConn1 -- Controlled Voltage Source/RConn2
  Current Sensor/LConn1 -- _RC1/LConn1 -- _R1/LConn1 -- u_cap/LConn1
  Current Sensor1/RConn2 -- _L1/RConn1
  _R1/RConn1 -- _L1/LConn1

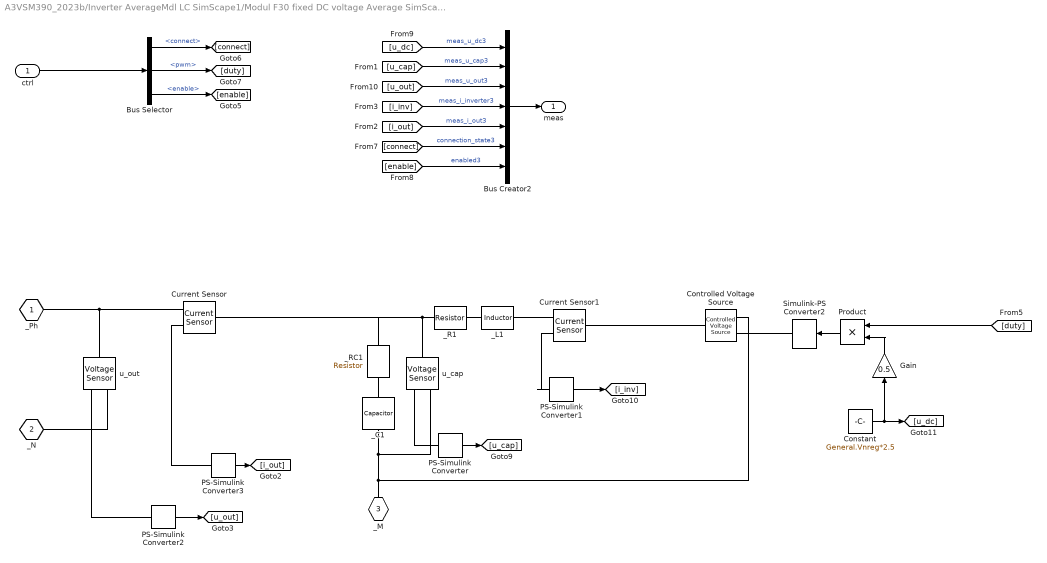
== system A3VSM390_2023b/Inverter AverageMdl LC SimScape1/Modul F30 fixed DC voltage Average SimScape/simscape_bridgefilter_aca2 ==
  ctrl : Inport
  Bus Creator2 : BusCreator  Inputs=7
  Bus Selector : BusSelector  OutputSignals=connect,pwm,enable
  Constant : Constant  Value=General.Vnreg*2.5
  Controlled Voltage Source : fl_lib/Electrical/Electrical Sources/Controlled Voltage Source
  Current Sensor : fl_lib/Electrical/Electrical Sensors/Current Sensor
  Current Sensor1 : fl_lib/Electrical/Electrical Sensors/Current Sensor
  Gain : Gain  Gain=0.5
  PS-Simulink Converter{,1..3} (4 alike) : nesl_utility/PS-Simulink Converter  PhysicalDomain=network_engine_domain  SubClassName=ps_output  LeftPortType=input  RightPortType=output  PseudoPeriodic=off  Frequencies=[]  VectorFormat=1-D array  Unit=1  AffineConversion=off
  Product : Product
  Simulink-PS Converter2 : nesl_utility/Simulink-PS Converter  PhysicalDomain=network_engine_domain  SubClassName=ps_input  LeftPortType=input  RightPortType=output  PseudoPeriodic=off  Frequencies=[]  NoiseDistribution=none  NoiseParameters=[]  Unit=1  AffineConversion=off  FilteringAndDerivatives=zero  SimscapeFilterOrder=1  InputFilterTimeConstant=0.001  UdotUserProvided=1
  _C1 : fl_lib/Electrical/Electrical Elements/Capacitor  c=C1 F  r=1e-6 Ohm  g=0 1/Ohm  i_specify=off  i_priority=None  i=0 A  i_nominal_specify=off  i_nominal_unit=A  i_nominal_value=1  v_specify=off  v_priority=None  v=0 V  v_nominal_specify=off  v_nominal_unit=V  v_nominal_value=1  vc_specify=off  vc_priority=None  vc=0 V  vc_nominal_specify=off  vc_nominal_unit=V  vc_nominal_value=1
  _L1 : fl_lib/Electrical/Electrical Elements/Inductor  l=L1 H  r=0 Ohm  g=1e-9 1/Ohm  i_specify=off  i_priority=None  i=0 A  i_nominal_specify=off  i_nominal_unit=A  i_nominal_value=1  v_specify=off  v_priority=None  v=0 V  v_nominal_specify=off  v_nominal_unit=V  v_nominal_value=1  i_L_specify=off  i_L_priority=None  i_L=0 A  i_L_nominal_specify=off  i_L_nominal_unit=A  i_L_nominal_value=1
  _R1 : fl_lib/Electrical/Electrical Elements/Resistor  R=R_L1 Ohm  i_specify=off  i_priority=None  i=0 A  i_nominal_specify=off  i_nominal_unit=A  i_nominal_value=1  v_specify=off  v_priority=None  v=0 V  v_nominal_specify=off  v_nominal_unit=V  v_nominal_value=1
  _RC1 : fl_lib/Electrical/Electrical Elements/Resistor  R=R_C1 Ohm  i_specify=off  i_priority=None  i=0 A  i_nominal_specify=off  i_nominal_unit=A  i_nominal_value=1  v_specify=off  v_priority=None  v=0 V  v_nominal_specify=off  v_nominal_unit=V  v_nominal_value=1
  u_cap : fl_lib/Electrical/Electrical Sensors/Voltage Sensor
  u_out : fl_lib/Electrical/Electrical Sensors/Voltage Sensor
  _Ph : PMIOPort  Side=Left
  _N : PMIOPort  Port=2  Side=Left
  _M : PMIOPort  Port=3  Side=Right
  meas : Outport  VectorParamsAs1DForOutWhenUnconnected=off
  wires:
  Bus Selector/2 -> [duty]  "<pwm>"
  Bus Selector/1 -> [connect]  "<connect>"
  [connect] -> Bus Creator2/6  "connection_state3"
  ctrl/1 -> Bus Selector/1
  [i_out] -> Bus Creator2/5  "meas_i_out3"
  [i_inv] -> Bus Creator2/4  "meas_i_inverter3"
  [u_out] -> Bus Creator2/3  "meas_u_out3"
  [u_cap] -> Bus Creator2/2  "meas_u_cap3"
  Bus Selector/3 -> [enable]  "<enable>"
  [enable] -> Bus Creator2/7  "enabled3"
  Bus Creator2/1 -> meas/1
  [u_dc] -> Bus Creator2/1  "meas_u_dc3"
  PS-Simulink Converter/1 -> [u_cap]
  PS-Simulink Converter1/1 -> [i_inv]
  PS-Simulink Converter2/1 -> [u_out]
  PS-Simulink Converter3/1 -> [i_out]
  Product/1 -> Simulink-PS Converter2/1
  Constant/1 -> [u_dc], Gain/1
  [duty] -> Product/1
  Gain/1 -> Product/2
  connections:
  _R1/RConn1 -- _L1/LConn1
  Current Sensor1/RConn2 -- _L1/RConn1
  u_cap/LConn1 -- _R1/LConn1 -- _RC1/LConn1 -- Current Sensor/LConn1
  Controlled Voltage Source/RConn2 -- _M/RConn1 -- u_cap/RConn2 -- _C1/RConn1
  u_out/LConn1 -- _Ph/RConn1 -- Current Sensor/RConn2
  u_out/RConn2 -- _N/RConn1
  Current Sensor1/LConn1 -- Controlled Voltage Source/LConn1
  Simulink-PS Converter2/RConn1 -- Controlled Voltage Source/RConn1
  PS-Simulink Converter/LConn1 -- u_cap/RConn1
  PS-Simulink Converter1/LConn1 -- Current Sensor1/RConn1
  PS-Simulink Converter2/LConn1 -- u_out/RConn1
  PS-Simulink Converter3/LConn1 -- Current Sensor/RConn1
  _RC1/RConn1 -- _C1/LConn1
